simulink subsystem "Open_Loop_Angle"  (R2024b)
settings: Solver=VariableStepAuto  StartTime=0.0  StopTime=10.0  RelTol=1e-3
libraries: simulink x1
settings Model: Creator=luigi  LastModifiedBy=luigi

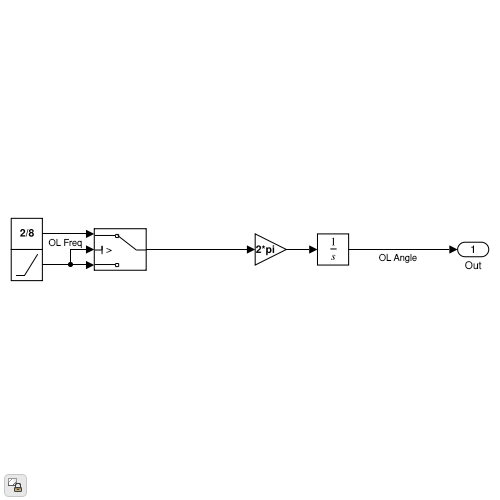
[thumbnail: Simulink's stored preview of the top-level diagram]
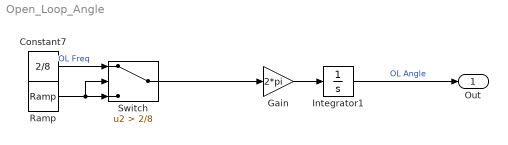
== system Open_Loop_Angle ==
  Constant7 : Constant  Value=2/8
  Gain : Gain  Gain=2*pi
  Integrator1 : Integrator
  Ramp : simulink/Sources/Ramp  slope=2/(8)  start=0  InitialOutput=0
  Switch : Switch  Criteria=u2 > Threshold  Threshold=2/8  SaturateOnIntegerOverflow=off  InputSameDT=off
  Out : Outport
  wires:
  Ramp/1 -> Switch/3, Switch/2
  Integrator1/1 -> Out/1  "OL Angle"
  Gain/1 -> Integrator1/1
  Constant7/1 -> Switch/1  "OL Freq"
  Switch/1 -> Gain/1
